simulink model "HSX_16_model - 복사본"  (R2023b)
settings: Solver=VariableStepAuto  StartTime=0.0  StopTime=30  RelTol=1e-3
undefined symbols (not defined in the file): LHSX, Ra, RHSX, Tsamp, Vf
libraries: spsControlledVoltageSourceLib x16, spsDCMachineLib x16, spsVoltageMeasurementLib x16, spsSeriesRLCBranchLib x2, spsCurrentMeasurementLib x1, spsGroundLib x1, spsIdealSwitchLib x1, sps_lib x1
settings Model: Creator=baik3-ad  LastModifiedBy=baik3-ad

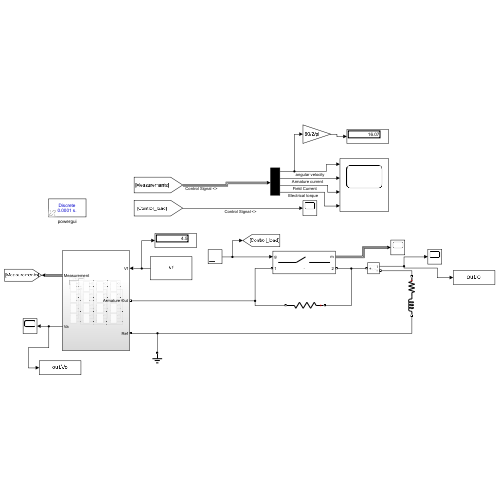
[thumbnail: Simulink's stored preview of the top-level diagram]
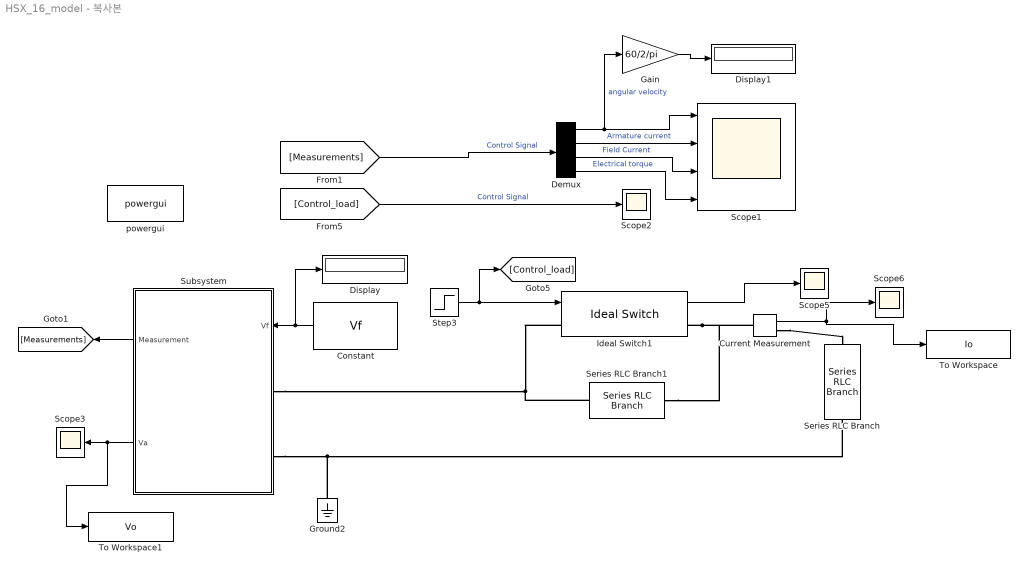
== system HSX_16_model - 복사본 ==
  Constant : Constant  Value=Vf
  Current Measurement : spsCurrentMeasurementLib/Current Measurement  PhasorSimulation=off  OutputType=Complex  PSBequivalent=0
  Demux : Demux
  Display : Display
  Display1 : Display
  Gain : Gain  Gain=60/2/pi
  Ground2 : spsGroundLib/Ground  LConnTagsString=a
  Ideal Switch1 : spsIdealSwitchLib/Ideal Switch  Ron=0.00001  Lon=0  IC=0  Rs=inf  Cs=0  Measurements=on
  Scope1 : Scope  NumInputPorts=4
  Scope{2..3,5..6} (4 alike) : Scope
  Series RLC Branch : spsSeriesRLCBranchLib/Series RLC Branch  LConnTagsString=__new0  RConnTagsString=__new0  BranchType=RL  Resistance=RHSX  Inductance=LHSX  SetiL0=off  InitialCurrent=0  Capacitance=1e-6  Setx0=off  InitialVoltage=0  Measurements=None
  Series RLC Branch1 : spsSeriesRLCBranchLib/Series RLC Branch  LConnTagsString=__new0  RConnTagsString=__new0  BranchType=R  Resistance=1e8  Inductance=LHSX  SetiL0=off  InitialCurrent=0  Capacitance=1e-6  Setx0=off  InitialVoltage=0  Measurements=None
  Step3 : Step  Time=12  SampleTime=0  VectorParams1D=off  ZeroCross=off
  Subsystem : Subsystem
  To Workspace : ToWorkspace  VariableName=Io  SaveFormat=Timeseries  SampleTime=-1
  To Workspace1 : ToWorkspace  VariableName=Vo  SaveFormat=Timeseries  SampleTime=-1
  powergui : sps_lib/powergui  Priority=1  SimulationMode=Discrete  SampleTime=Tsamp  frequency=60  Iterations=50  frequencyindice=0  Pbase=100e6  ErrMax=1e-4  UnitsV=kV  UnitsW=MW  buscounter=0  FunctionMessages=off  echomessages=off  EnableUseOfTLC=off  CurrentSourceSwitches=off  DisableSnubberDevices=off  DisableRonSwitches=off  DisableVfSwitches=off  DisplayEquations=off  AutomaticDiscreteSolvers=off  SolverType=Tustin/Backward Euler (TBE)  Interpol=off  ExternalGateDelay=off  methode=off  Ts=100  x0status=blocks  SPID=on  SwTol=0  HookPort=off  NonlinearTolerance=1e-4  nMaxIteration=100  ContinueOnMaxIteration=off  RestoreLinks=warning  ResistiveCurrentMeasurement=off  Frange=[0:2:500]  Ylog=off  Xlog=on  ShowGrid=off  save=off  variable=ZData  structure=0  ZoomFFT=off  StartTime=0.0  cycles=1  DisplayStyle=1  fundamental=60  FreqAxis=off  MaxFrequency=1000  frequencyindicesteady=1  RmsSteady=1  display=off
  wires:
  Current Measurement/1 -> To Workspace/1, Scope6/1
  Step3/1 -> [Control_load], Ideal Switch1/1
  Ideal Switch1/1 -> Scope5/1
  Constant/1 -> Display/1, Subsystem/1(Vf)
  [Control_load] -> Scope2/1  "Control Signal"
  Subsystem/1(Measurement) -> [Measurements]
  [Measurements] -> Demux/1  "Control Signal"
  Subsystem/2(Va) -> To Workspace1/1, Scope3/1
  Demux/1 -> Gain/1, Scope1/1  "angular velocity"
  Demux/2 -> Scope1/2  "Armature current"
  Demux/3 -> Scope1/3  "Field Current"
  Demux/4 -> Scope1/4  "Electrical torque"
  Gain/1 -> Display1/1
  connections:
  Ideal Switch1/RConn1 -- Series RLC Branch1/LConn1 -- Current Measurement/LConn1
  Ideal Switch1/LConn1 -- Series RLC Branch1/RConn1 -- Subsystem/LConn1
  Current Measurement/RConn1 -- Series RLC Branch/LConn1
  Ground2/LConn1 -- Subsystem/LConn2 -- Series RLC Branch/RConn1

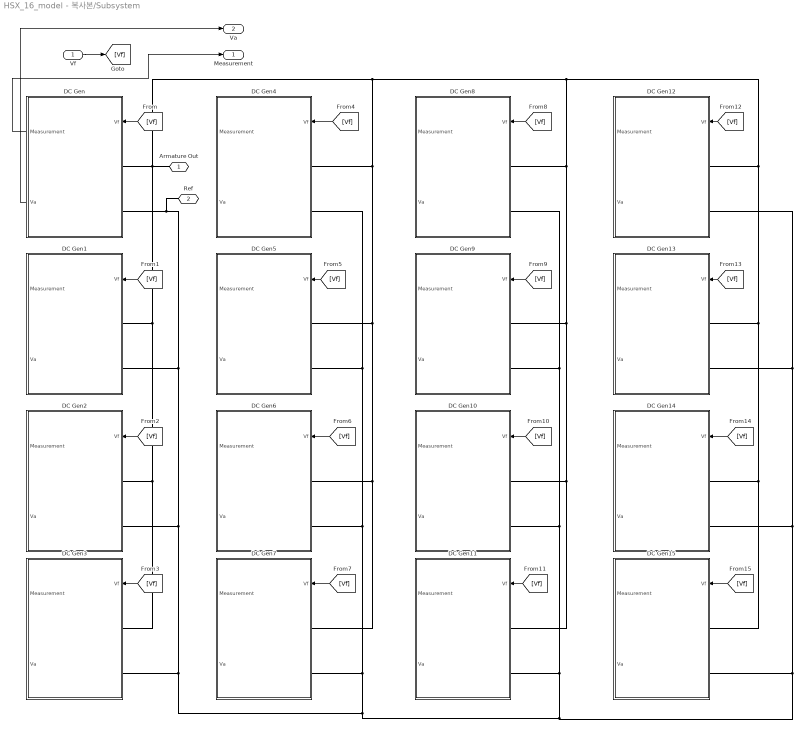
== system HSX_16_model - 복사본/Subsystem ==
  Vf : Inport
  DC Gen : Subsystem
  DC Gen1 : Subsystem
  DC Gen10 : Subsystem
  DC Gen11 : Subsystem
  DC Gen12 : Subsystem
  DC Gen13 : Subsystem
  DC Gen14 : Subsystem
  DC Gen15 : Subsystem
  DC Gen2 : Subsystem
  DC Gen3 : Subsystem
  DC Gen4 : Subsystem
  DC Gen5 : Subsystem
  DC Gen6 : Subsystem
  DC Gen7 : Subsystem
  DC Gen8 : Subsystem
  DC Gen9 : Subsystem
  Armature Out : PMIOPort  Side=Left
  Ref : PMIOPort  Port=2  Side=Left
  Measurement : Outport
  Va : Outport  Port=2
  wires:
  Vf/1 -> [Vf]
  [Vf] -> DC Gen/1(Vf)
  [Vf] -> DC Gen1/1(Vf)
  [Vf] -> DC Gen2/1(Vf)
  [Vf] -> DC Gen3/1(Vf)
  [Vf] -> DC Gen4/1(Vf)
  [Vf] -> DC Gen5/1(Vf)
  [Vf] -> DC Gen6/1(Vf)
  [Vf] -> DC Gen7/1(Vf)
  [Vf] -> DC Gen8/1(Vf)
  [Vf] -> DC Gen9/1(Vf)
  [Vf] -> DC Gen10/1(Vf)
  [Vf] -> DC Gen11/1(Vf)
  [Vf] -> DC Gen12/1(Vf)
  [Vf] -> DC Gen13/1(Vf)
  [Vf] -> DC Gen14/1(Vf)
  [Vf] -> DC Gen15/1(Vf)
  DC Gen/1(Measurement) -> Measurement/1
  DC Gen/2(Va) -> Va/1
  connections:
  Armature Out/RConn1 -- DC Gen1/LConn1 -- DC Gen2/LConn1 -- DC Gen3/LConn1 -- DC Gen15/LConn1 -- DC Gen14/LConn1 -- DC Gen13/LConn1 -- DC Gen12/LConn1 -- DC Gen11/LConn1 -- DC Gen10/LConn1 -- DC Gen9/LConn1 -- DC Gen8/LConn1 -- DC Gen7/LConn1 -- DC Gen6/LConn1 -- DC Gen5/LConn1 -- DC Gen4/LConn1 -- DC Gen/LConn1
  DC Gen/LConn2 -- DC Gen2/LConn2 -- DC Gen15/LConn2 -- DC Gen12/LConn2 -- DC Gen13/LConn2 -- DC Gen14/LConn2 -- DC Gen8/LConn2 -- DC Gen9/LConn2 -- DC Gen10/LConn2 -- DC Gen11/LConn2 -- DC Gen4/LConn2 -- DC Gen5/LConn2 -- DC Gen6/LConn2 -- DC Gen7/LConn2 -- DC Gen3/LConn2 -- DC Gen1/LConn2 -- Ref/RConn1

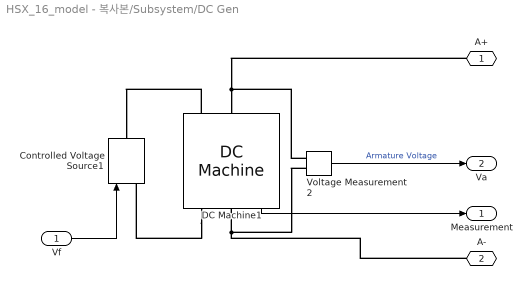
== system HSX_16_model - 복사본/Subsystem/DC Gen ==
  Vf : Inport
  Controlled Voltage Source1 : spsControlledVoltageSourceLib/Controlled Voltage Source  Initialize=on  Source_Type=DC  Amplitude=0  Phase=0  Frequency=0  Measurements=Voltage
  DC Machine1 : spsDCMachineLib/DC Machine  PresetModel=No  MechanicalLoad=Torque TL  FieldType=Wound  ShowDetailedParameters=on  MeasurementBus=off  RLa="[Ra  0.002]"  RLf=[0.0054 0.0125]  Laf=Laf  MachineConstant=Torque constant (N.m/A)  Ke=1.8  Kt=1.8  J=137  Bm=0  Tf=0  w0=w_initial  Ifinit=0  TsPowergui=0  TsBlock=-1
  Voltage Measurement2 : spsVoltageMeasurementLib/Voltage Measurement  PhasorSimulation=off  OutputType=Complex  PSBequivalent=0
  A+ : PMIOPort  Side=Left
  A- : PMIOPort  Port=2  Side=Left
  Measurement : Outport
  Va : Outport  Port=2
  wires:
  DC Machine1/1 -> Measurement/1
  Vf/1 -> Controlled Voltage Source1/1
  Voltage Measurement2/1 -> Va/1  "Armature Voltage"
  connections:
  Voltage Measurement2/LConn1 -- A+/RConn1 -- DC Machine1/LConn1
  Voltage Measurement2/LConn2 -- A-/RConn1 -- DC Machine1/RConn1
  DC Machine1/LConn2 -- Controlled Voltage Source1/RConn1
  DC Machine1/RConn2 -- Controlled Voltage Source1/LConn1

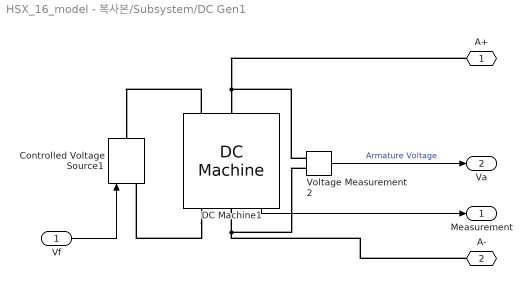
== system HSX_16_model - 복사본/Subsystem/DC Gen1 ==
  Vf : Inport
  Controlled Voltage Source1 : spsControlledVoltageSourceLib/Controlled Voltage Source  Initialize=on  Source_Type=DC  Amplitude=0  Phase=0  Frequency=0  Measurements=Voltage
  DC Machine1 : spsDCMachineLib/DC Machine  PresetModel=No  MechanicalLoad=Torque TL  FieldType=Wound  ShowDetailedParameters=on  MeasurementBus=off  RLa="[Ra  0.002]"  RLf=[0.0054 0.0125]  Laf=Laf  MachineConstant=Torque constant (N.m/A)  Ke=1.8  Kt=1.8  J=137  Bm=0  Tf=0  w0=w_initial  Ifinit=0  TsPowergui=0  TsBlock=-1
  Voltage Measurement2 : spsVoltageMeasurementLib/Voltage Measurement  PhasorSimulation=off  OutputType=Complex  PSBequivalent=0
  A+ : PMIOPort  Side=Left
  A- : PMIOPort  Port=2  Side=Left
  Measurement : Outport
  Va : Outport  Port=2
  wires:
  DC Machine1/1 -> Measurement/1
  Vf/1 -> Controlled Voltage Source1/1
  Voltage Measurement2/1 -> Va/1  "Armature Voltage"
  connections:
  Voltage Measurement2/LConn1 -- A+/RConn1 -- DC Machine1/LConn1
  Voltage Measurement2/LConn2 -- A-/RConn1 -- DC Machine1/RConn1
  DC Machine1/LConn2 -- Controlled Voltage Source1/RConn1
  DC Machine1/RConn2 -- Controlled Voltage Source1/LConn1

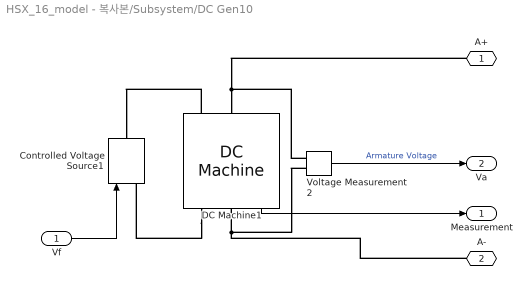
== system HSX_16_model - 복사본/Subsystem/DC Gen10 ==
  Vf : Inport
  Controlled Voltage Source1 : spsControlledVoltageSourceLib/Controlled Voltage Source  Initialize=on  Source_Type=DC  Amplitude=0  Phase=0  Frequency=0  Measurements=Voltage
  DC Machine1 : spsDCMachineLib/DC Machine  PresetModel=No  MechanicalLoad=Torque TL  FieldType=Wound  ShowDetailedParameters=on  MeasurementBus=off  RLa="[Ra  0.002]"  RLf=[0.0054 0.0125]  Laf=Laf  MachineConstant=Torque constant (N.m/A)  Ke=1.8  Kt=1.8  J=137  Bm=0  Tf=0  w0=w_initial  Ifinit=0  TsPowergui=0  TsBlock=-1
  Voltage Measurement2 : spsVoltageMeasurementLib/Voltage Measurement  PhasorSimulation=off  OutputType=Complex  PSBequivalent=0
  A+ : PMIOPort  Side=Left
  A- : PMIOPort  Port=2  Side=Left
  Measurement : Outport
  Va : Outport  Port=2
  wires:
  DC Machine1/1 -> Measurement/1
  Vf/1 -> Controlled Voltage Source1/1
  Voltage Measurement2/1 -> Va/1  "Armature Voltage"
  connections:
  Voltage Measurement2/LConn1 -- A+/RConn1 -- DC Machine1/LConn1
  Voltage Measurement2/LConn2 -- A-/RConn1 -- DC Machine1/RConn1
  DC Machine1/LConn2 -- Controlled Voltage Source1/RConn1
  DC Machine1/RConn2 -- Controlled Voltage Source1/LConn1

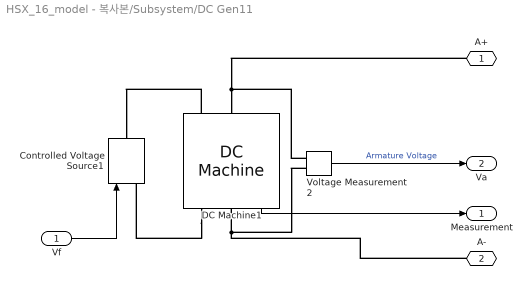
== system HSX_16_model - 복사본/Subsystem/DC Gen11 ==
  Vf : Inport
  Controlled Voltage Source1 : spsControlledVoltageSourceLib/Controlled Voltage Source  Initialize=on  Source_Type=DC  Amplitude=0  Phase=0  Frequency=0  Measurements=Voltage
  DC Machine1 : spsDCMachineLib/DC Machine  PresetModel=No  MechanicalLoad=Torque TL  FieldType=Wound  ShowDetailedParameters=on  MeasurementBus=off  RLa="[Ra  0.002]"  RLf=[0.0054 0.0125]  Laf=Laf  MachineConstant=Torque constant (N.m/A)  Ke=1.8  Kt=1.8  J=137  Bm=0  Tf=0  w0=w_initial  Ifinit=0  TsPowergui=0  TsBlock=-1
  Voltage Measurement2 : spsVoltageMeasurementLib/Voltage Measurement  PhasorSimulation=off  OutputType=Complex  PSBequivalent=0
  A+ : PMIOPort  Side=Left
  A- : PMIOPort  Port=2  Side=Left
  Measurement : Outport
  Va : Outport  Port=2
  wires:
  DC Machine1/1 -> Measurement/1
  Vf/1 -> Controlled Voltage Source1/1
  Voltage Measurement2/1 -> Va/1  "Armature Voltage"
  connections:
  Voltage Measurement2/LConn1 -- A+/RConn1 -- DC Machine1/LConn1
  Voltage Measurement2/LConn2 -- A-/RConn1 -- DC Machine1/RConn1
  DC Machine1/LConn2 -- Controlled Voltage Source1/RConn1
  DC Machine1/RConn2 -- Controlled Voltage Source1/LConn1

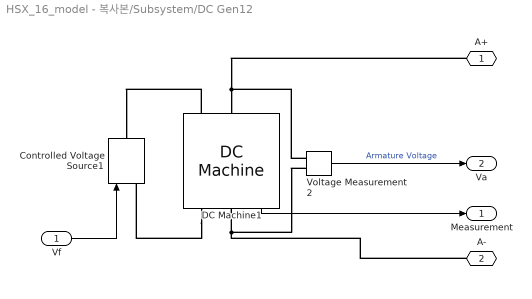
== system HSX_16_model - 복사본/Subsystem/DC Gen12 ==
  Vf : Inport
  Controlled Voltage Source1 : spsControlledVoltageSourceLib/Controlled Voltage Source  Initialize=on  Source_Type=DC  Amplitude=0  Phase=0  Frequency=0  Measurements=Voltage
  DC Machine1 : spsDCMachineLib/DC Machine  PresetModel=No  MechanicalLoad=Torque TL  FieldType=Wound  ShowDetailedParameters=on  MeasurementBus=off  RLa="[Ra  0.002]"  RLf=[0.0054 0.0125]  Laf=Laf  MachineConstant=Torque constant (N.m/A)  Ke=1.8  Kt=1.8  J=137  Bm=0  Tf=0  w0=w_initial  Ifinit=0  TsPowergui=0  TsBlock=-1
  Voltage Measurement2 : spsVoltageMeasurementLib/Voltage Measurement  PhasorSimulation=off  OutputType=Complex  PSBequivalent=0
  A+ : PMIOPort  Side=Left
  A- : PMIOPort  Port=2  Side=Left
  Measurement : Outport
  Va : Outport  Port=2
  wires:
  DC Machine1/1 -> Measurement/1
  Vf/1 -> Controlled Voltage Source1/1
  Voltage Measurement2/1 -> Va/1  "Armature Voltage"
  connections:
  Voltage Measurement2/LConn1 -- A+/RConn1 -- DC Machine1/LConn1
  Voltage Measurement2/LConn2 -- A-/RConn1 -- DC Machine1/RConn1
  DC Machine1/LConn2 -- Controlled Voltage Source1/RConn1
  DC Machine1/RConn2 -- Controlled Voltage Source1/LConn1

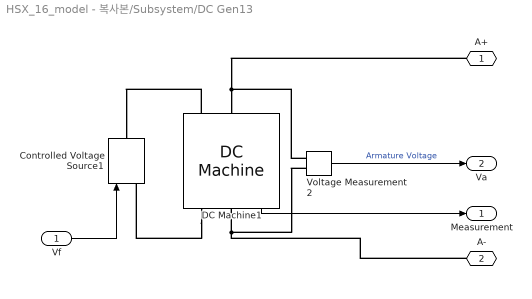
== system HSX_16_model - 복사본/Subsystem/DC Gen13 ==
  Vf : Inport
  Controlled Voltage Source1 : spsControlledVoltageSourceLib/Controlled Voltage Source  Initialize=on  Source_Type=DC  Amplitude=0  Phase=0  Frequency=0  Measurements=Voltage
  DC Machine1 : spsDCMachineLib/DC Machine  PresetModel=No  MechanicalLoad=Torque TL  FieldType=Wound  ShowDetailedParameters=on  MeasurementBus=off  RLa="[Ra  0.002]"  RLf=[0.0054 0.0125]  Laf=Laf  MachineConstant=Torque constant (N.m/A)  Ke=1.8  Kt=1.8  J=137  Bm=0  Tf=0  w0=w_initial  Ifinit=0  TsPowergui=0  TsBlock=-1
  Voltage Measurement2 : spsVoltageMeasurementLib/Voltage Measurement  PhasorSimulation=off  OutputType=Complex  PSBequivalent=0
  A+ : PMIOPort  Side=Left
  A- : PMIOPort  Port=2  Side=Left
  Measurement : Outport
  Va : Outport  Port=2
  wires:
  DC Machine1/1 -> Measurement/1
  Vf/1 -> Controlled Voltage Source1/1
  Voltage Measurement2/1 -> Va/1  "Armature Voltage"
  connections:
  Voltage Measurement2/LConn1 -- A+/RConn1 -- DC Machine1/LConn1
  Voltage Measurement2/LConn2 -- A-/RConn1 -- DC Machine1/RConn1
  DC Machine1/LConn2 -- Controlled Voltage Source1/RConn1
  DC Machine1/RConn2 -- Controlled Voltage Source1/LConn1

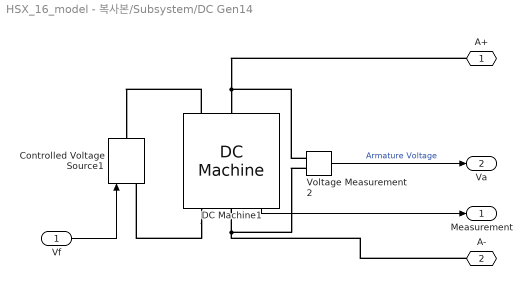
== system HSX_16_model - 복사본/Subsystem/DC Gen14 ==
  Vf : Inport
  Controlled Voltage Source1 : spsControlledVoltageSourceLib/Controlled Voltage Source  Initialize=on  Source_Type=DC  Amplitude=0  Phase=0  Frequency=0  Measurements=Voltage
  DC Machine1 : spsDCMachineLib/DC Machine  PresetModel=No  MechanicalLoad=Torque TL  FieldType=Wound  ShowDetailedParameters=on  MeasurementBus=off  RLa="[Ra  0.002]"  RLf=[0.0054 0.0125]  Laf=Laf  MachineConstant=Torque constant (N.m/A)  Ke=1.8  Kt=1.8  J=137  Bm=0  Tf=0  w0=w_initial  Ifinit=0  TsPowergui=0  TsBlock=-1
  Voltage Measurement2 : spsVoltageMeasurementLib/Voltage Measurement  PhasorSimulation=off  OutputType=Complex  PSBequivalent=0
  A+ : PMIOPort  Side=Left
  A- : PMIOPort  Port=2  Side=Left
  Measurement : Outport
  Va : Outport  Port=2
  wires:
  DC Machine1/1 -> Measurement/1
  Vf/1 -> Controlled Voltage Source1/1
  Voltage Measurement2/1 -> Va/1  "Armature Voltage"
  connections:
  Voltage Measurement2/LConn1 -- A+/RConn1 -- DC Machine1/LConn1
  Voltage Measurement2/LConn2 -- A-/RConn1 -- DC Machine1/RConn1
  DC Machine1/LConn2 -- Controlled Voltage Source1/RConn1
  DC Machine1/RConn2 -- Controlled Voltage Source1/LConn1

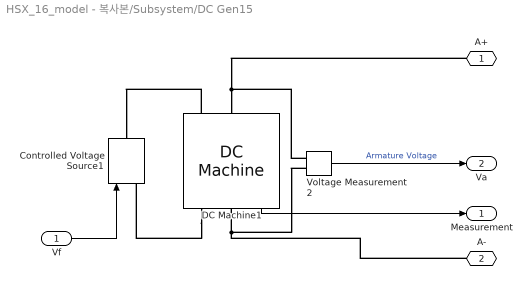
== system HSX_16_model - 복사본/Subsystem/DC Gen15 ==
  Vf : Inport
  Controlled Voltage Source1 : spsControlledVoltageSourceLib/Controlled Voltage Source  Initialize=on  Source_Type=DC  Amplitude=0  Phase=0  Frequency=0  Measurements=Voltage
  DC Machine1 : spsDCMachineLib/DC Machine  PresetModel=No  MechanicalLoad=Torque TL  FieldType=Wound  ShowDetailedParameters=on  MeasurementBus=off  RLa="[Ra  0.002]"  RLf=[0.0054 0.0125]  Laf=Laf  MachineConstant=Torque constant (N.m/A)  Ke=1.8  Kt=1.8  J=137  Bm=0  Tf=0  w0=w_initial  Ifinit=0  TsPowergui=0  TsBlock=-1
  Voltage Measurement2 : spsVoltageMeasurementLib/Voltage Measurement  PhasorSimulation=off  OutputType=Complex  PSBequivalent=0
  A+ : PMIOPort  Side=Left
  A- : PMIOPort  Port=2  Side=Left
  Measurement : Outport
  Va : Outport  Port=2
  wires:
  DC Machine1/1 -> Measurement/1
  Vf/1 -> Controlled Voltage Source1/1
  Voltage Measurement2/1 -> Va/1  "Armature Voltage"
  connections:
  Voltage Measurement2/LConn1 -- A+/RConn1 -- DC Machine1/LConn1
  Voltage Measurement2/LConn2 -- A-/RConn1 -- DC Machine1/RConn1
  DC Machine1/LConn2 -- Controlled Voltage Source1/RConn1
  DC Machine1/RConn2 -- Controlled Voltage Source1/LConn1

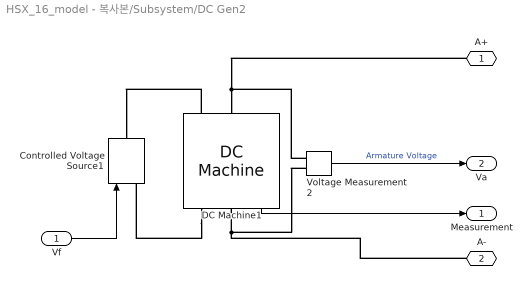
== system HSX_16_model - 복사본/Subsystem/DC Gen2 ==
  Vf : Inport
  Controlled Voltage Source1 : spsControlledVoltageSourceLib/Controlled Voltage Source  Initialize=on  Source_Type=DC  Amplitude=0  Phase=0  Frequency=0  Measurements=Voltage
  DC Machine1 : spsDCMachineLib/DC Machine  PresetModel=No  MechanicalLoad=Torque TL  FieldType=Wound  ShowDetailedParameters=on  MeasurementBus=off  RLa="[Ra  0.002]"  RLf=[0.0054 0.0125]  Laf=Laf  MachineConstant=Torque constant (N.m/A)  Ke=1.8  Kt=1.8  J=137  Bm=0  Tf=0  w0=w_initial  Ifinit=0  TsPowergui=0  TsBlock=-1
  Voltage Measurement2 : spsVoltageMeasurementLib/Voltage Measurement  PhasorSimulation=off  OutputType=Complex  PSBequivalent=0
  A+ : PMIOPort  Side=Left
  A- : PMIOPort  Port=2  Side=Left
  Measurement : Outport
  Va : Outport  Port=2
  wires:
  DC Machine1/1 -> Measurement/1
  Vf/1 -> Controlled Voltage Source1/1
  Voltage Measurement2/1 -> Va/1  "Armature Voltage"
  connections:
  Voltage Measurement2/LConn1 -- A+/RConn1 -- DC Machine1/LConn1
  Voltage Measurement2/LConn2 -- A-/RConn1 -- DC Machine1/RConn1
  DC Machine1/LConn2 -- Controlled Voltage Source1/RConn1
  DC Machine1/RConn2 -- Controlled Voltage Source1/LConn1

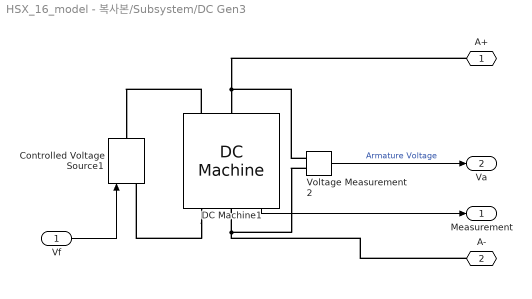
== system HSX_16_model - 복사본/Subsystem/DC Gen3 ==
  Vf : Inport
  Controlled Voltage Source1 : spsControlledVoltageSourceLib/Controlled Voltage Source  Initialize=on  Source_Type=DC  Amplitude=0  Phase=0  Frequency=0  Measurements=Voltage
  DC Machine1 : spsDCMachineLib/DC Machine  PresetModel=No  MechanicalLoad=Torque TL  FieldType=Wound  ShowDetailedParameters=on  MeasurementBus=off  RLa="[Ra  0.002]"  RLf=[0.0054 0.0125]  Laf=Laf  MachineConstant=Torque constant (N.m/A)  Ke=1.8  Kt=1.8  J=137  Bm=0  Tf=0  w0=w_initial  Ifinit=0  TsPowergui=0  TsBlock=-1
  Voltage Measurement2 : spsVoltageMeasurementLib/Voltage Measurement  PhasorSimulation=off  OutputType=Complex  PSBequivalent=0
  A+ : PMIOPort  Side=Left
  A- : PMIOPort  Port=2  Side=Left
  Measurement : Outport
  Va : Outport  Port=2
  wires:
  DC Machine1/1 -> Measurement/1
  Vf/1 -> Controlled Voltage Source1/1
  Voltage Measurement2/1 -> Va/1  "Armature Voltage"
  connections:
  Voltage Measurement2/LConn1 -- A+/RConn1 -- DC Machine1/LConn1
  Voltage Measurement2/LConn2 -- A-/RConn1 -- DC Machine1/RConn1
  DC Machine1/LConn2 -- Controlled Voltage Source1/RConn1
  DC Machine1/RConn2 -- Controlled Voltage Source1/LConn1

== system HSX_16_model - 복사본/Subsystem/DC Gen4 ==
  Vf : Inport
  Controlled Voltage Source1 : spsControlledVoltageSourceLib/Controlled Voltage Source  Initialize=on  Source_Type=DC  Amplitude=0  Phase=0  Frequency=0  Measurements=Voltage
  DC Machine1 : spsDCMachineLib/DC Machine  PresetModel=No  MechanicalLoad=Torque TL  FieldType=Wound  ShowDetailedParameters=on  MeasurementBus=off  RLa="[Ra  0.002]"  RLf=[0.0054 0.0125]  Laf=Laf  MachineConstant=Torque constant (N.m/A)  Ke=1.8  Kt=1.8  J=137  Bm=0  Tf=0  w0=w_initial  Ifinit=0  TsPowergui=0  TsBlock=-1
  Voltage Measurement2 : spsVoltageMeasurementLib/Voltage Measurement  PhasorSimulation=off  OutputType=Complex  PSBequivalent=0
  A+ : PMIOPort  Side=Left
  A- : PMIOPort  Port=2  Side=Left
  Measurement : Outport
  Va : Outport  Port=2
  wires:
  DC Machine1/1 -> Measurement/1
  Vf/1 -> Controlled Voltage Source1/1
  Voltage Measurement2/1 -> Va/1  "Armature Voltage"
  connections:
  Voltage Measurement2/LConn1 -- A+/RConn1 -- DC Machine1/LConn1
  Voltage Measurement2/LConn2 -- A-/RConn1 -- DC Machine1/RConn1
  DC Machine1/LConn2 -- Controlled Voltage Source1/RConn1
  DC Machine1/RConn2 -- Controlled Voltage Source1/LConn1

== system HSX_16_model - 복사본/Subsystem/DC Gen5 ==
  Vf : Inport
  Controlled Voltage Source1 : spsControlledVoltageSourceLib/Controlled Voltage Source  Initialize=on  Source_Type=DC  Amplitude=0  Phase=0  Frequency=0  Measurements=Voltage
  DC Machine1 : spsDCMachineLib/DC Machine  PresetModel=No  MechanicalLoad=Torque TL  FieldType=Wound  ShowDetailedParameters=on  MeasurementBus=off  RLa="[Ra  0.002]"  RLf=[0.0054 0.0125]  Laf=Laf  MachineConstant=Torque constant (N.m/A)  Ke=1.8  Kt=1.8  J=137  Bm=0  Tf=0  w0=w_initial  Ifinit=0  TsPowergui=0  TsBlock=-1
  Voltage Measurement2 : spsVoltageMeasurementLib/Voltage Measurement  PhasorSimulation=off  OutputType=Complex  PSBequivalent=0
  A+ : PMIOPort  Side=Left
  A- : PMIOPort  Port=2  Side=Left
  Measurement : Outport
  Va : Outport  Port=2
  wires:
  DC Machine1/1 -> Measurement/1
  Vf/1 -> Controlled Voltage Source1/1
  Voltage Measurement2/1 -> Va/1  "Armature Voltage"
  connections:
  Voltage Measurement2/LConn1 -- A+/RConn1 -- DC Machine1/LConn1
  Voltage Measurement2/LConn2 -- A-/RConn1 -- DC Machine1/RConn1
  DC Machine1/LConn2 -- Controlled Voltage Source1/RConn1
  DC Machine1/RConn2 -- Controlled Voltage Source1/LConn1

== system HSX_16_model - 복사본/Subsystem/DC Gen6 ==
  Vf : Inport
  Controlled Voltage Source1 : spsControlledVoltageSourceLib/Controlled Voltage Source  Initialize=on  Source_Type=DC  Amplitude=0  Phase=0  Frequency=0  Measurements=Voltage
  DC Machine1 : spsDCMachineLib/DC Machine  PresetModel=No  MechanicalLoad=Torque TL  FieldType=Wound  ShowDetailedParameters=on  MeasurementBus=off  RLa="[Ra  0.002]"  RLf=[0.0054 0.0125]  Laf=Laf  MachineConstant=Torque constant (N.m/A)  Ke=1.8  Kt=1.8  J=137  Bm=0  Tf=0  w0=w_initial  Ifinit=0  TsPowergui=0  TsBlock=-1
  Voltage Measurement2 : spsVoltageMeasurementLib/Voltage Measurement  PhasorSimulation=off  OutputType=Complex  PSBequivalent=0
  A+ : PMIOPort  Side=Left
  A- : PMIOPort  Port=2  Side=Left
  Measurement : Outport
  Va : Outport  Port=2
  wires:
  DC Machine1/1 -> Measurement/1
  Vf/1 -> Controlled Voltage Source1/1
  Voltage Measurement2/1 -> Va/1  "Armature Voltage"
  connections:
  Voltage Measurement2/LConn1 -- A+/RConn1 -- DC Machine1/LConn1
  Voltage Measurement2/LConn2 -- A-/RConn1 -- DC Machine1/RConn1
  DC Machine1/LConn2 -- Controlled Voltage Source1/RConn1
  DC Machine1/RConn2 -- Controlled Voltage Source1/LConn1

== system HSX_16_model - 복사본/Subsystem/DC Gen7 ==
  Vf : Inport
  Controlled Voltage Source1 : spsControlledVoltageSourceLib/Controlled Voltage Source  Initialize=on  Source_Type=DC  Amplitude=0  Phase=0  Frequency=0  Measurements=Voltage
  DC Machine1 : spsDCMachineLib/DC Machine  PresetModel=No  MechanicalLoad=Torque TL  FieldType=Wound  ShowDetailedParameters=on  MeasurementBus=off  RLa="[Ra  0.002]"  RLf=[0.0054 0.0125]  Laf=Laf  MachineConstant=Torque constant (N.m/A)  Ke=1.8  Kt=1.8  J=137  Bm=0  Tf=0  w0=w_initial  Ifinit=0  TsPowergui=0  TsBlock=-1
  Voltage Measurement2 : spsVoltageMeasurementLib/Voltage Measurement  PhasorSimulation=off  OutputType=Complex  PSBequivalent=0
  A+ : PMIOPort  Side=Left
  A- : PMIOPort  Port=2  Side=Left
  Measurement : Outport
  Va : Outport  Port=2
  wires:
  DC Machine1/1 -> Measurement/1
  Vf/1 -> Controlled Voltage Source1/1
  Voltage Measurement2/1 -> Va/1  "Armature Voltage"
  connections:
  Voltage Measurement2/LConn1 -- A+/RConn1 -- DC Machine1/LConn1
  Voltage Measurement2/LConn2 -- A-/RConn1 -- DC Machine1/RConn1
  DC Machine1/LConn2 -- Controlled Voltage Source1/RConn1
  DC Machine1/RConn2 -- Controlled Voltage Source1/LConn1

== system HSX_16_model - 복사본/Subsystem/DC Gen8 ==
  Vf : Inport
  Controlled Voltage Source1 : spsControlledVoltageSourceLib/Controlled Voltage Source  Initialize=on  Source_Type=DC  Amplitude=0  Phase=0  Frequency=0  Measurements=Voltage
  DC Machine1 : spsDCMachineLib/DC Machine  PresetModel=No  MechanicalLoad=Torque TL  FieldType=Wound  ShowDetailedParameters=on  MeasurementBus=off  RLa="[Ra  0.002]"  RLf=[0.0054 0.0125]  Laf=Laf  MachineConstant=Torque constant (N.m/A)  Ke=1.8  Kt=1.8  J=137  Bm=0  Tf=0  w0=w_initial  Ifinit=0  TsPowergui=0  TsBlock=-1
  Voltage Measurement2 : spsVoltageMeasurementLib/Voltage Measurement  PhasorSimulation=off  OutputType=Complex  PSBequivalent=0
  A+ : PMIOPort  Side=Left
  A- : PMIOPort  Port=2  Side=Left
  Measurement : Outport
  Va : Outport  Port=2
  wires:
  DC Machine1/1 -> Measurement/1
  Vf/1 -> Controlled Voltage Source1/1
  Voltage Measurement2/1 -> Va/1  "Armature Voltage"
  connections:
  Voltage Measurement2/LConn1 -- A+/RConn1 -- DC Machine1/LConn1
  Voltage Measurement2/LConn2 -- A-/RConn1 -- DC Machine1/RConn1
  DC Machine1/LConn2 -- Controlled Voltage Source1/RConn1
  DC Machine1/RConn2 -- Controlled Voltage Source1/LConn1

== system HSX_16_model - 복사본/Subsystem/DC Gen9 ==
  Vf : Inport
  Controlled Voltage Source1 : spsControlledVoltageSourceLib/Controlled Voltage Source  Initialize=on  Source_Type=DC  Amplitude=0  Phase=0  Frequency=0  Measurements=Voltage
  DC Machine1 : spsDCMachineLib/DC Machine  PresetModel=No  MechanicalLoad=Torque TL  FieldType=Wound  ShowDetailedParameters=on  MeasurementBus=off  RLa="[Ra  0.002]"  RLf=[0.0054 0.0125]  Laf=Laf  MachineConstant=Torque constant (N.m/A)  Ke=1.8  Kt=1.8  J=137  Bm=0  Tf=0  w0=w_initial  Ifinit=0  TsPowergui=0  TsBlock=-1
  Voltage Measurement2 : spsVoltageMeasurementLib/Voltage Measurement  PhasorSimulation=off  OutputType=Complex  PSBequivalent=0
  A+ : PMIOPort  Side=Left
  A- : PMIOPort  Port=2  Side=Left
  Measurement : Outport
  Va : Outport  Port=2
  wires:
  DC Machine1/1 -> Measurement/1
  Vf/1 -> Controlled Voltage Source1/1
  Voltage Measurement2/1 -> Va/1  "Armature Voltage"
  connections:
  Voltage Measurement2/LConn1 -- A+/RConn1 -- DC Machine1/LConn1
  Voltage Measurement2/LConn2 -- A-/RConn1 -- DC Machine1/RConn1
  DC Machine1/LConn2 -- Controlled Voltage Source1/RConn1
  DC Machine1/RConn2 -- Controlled Voltage Source1/LConn1
